simulink model "Swingup_LQR_energy_2021"  (R2021a)
settings: Solver=FixedStepAuto  StartTime=0.0  StopTime=100  RelTol=1e-3
PreLoadFcn:
  | waijung.modelPreload; % Required for working with Waijung Blockset. Do not remove.
undefined symbols (not defined in the file or in its folder): HSEOSC, Link, LQFP100, ST, STM32F407VG
libraries: simulink x2, stm32f4_io_lib x1, stm32f4_device_config_lib x1
CloseFcn:
  | waijung.modelClose; % Required for working with Waijung Blockset. Do not remove.
settings Model: Creator=MINH TAI  LastModifiedBy=NGAI-LAPTOP
settings SolverCC: AlgebraicLoopSolver=TrustRegion
settings DataIOCC: ReturnWorkspaceOutputs=off
settings OptimizationCC: DefaultParameterBehavior=Inlined  EnhancedBackFolding=on  PassReuseOutputArgsAs=Individual arguments  OptimizeBlockOrder=speed  DifferentSizesBufferReuse=on  OptimizationCustomize=off  EfficientTunableParamExpr=on
settings DebuggingCC: ParameterTunabilityLossMsg=error  SFMachineParentedDataDiag=warning  ArithmeticOperatorsInVariantConditions=warning
settings HardwareCC: ProdBitPerPointer=32  ProdBitPerSizeT=32  ProdBitPerPtrDiffT=32  ProdLargestAtomicFloat=None  ProdIntDivRoundTo=Undefined  ProdWordSize=32  ProdHWDeviceType=ARM Compatible->Cortex - M4  TargetEndianess=LittleEndian  TargetHWDeviceType=ARM Compatible->Cortex - M4
settings SFSimCC: SimUseLocalCustomCode=off  MATLABDynamicMemAlloc=off  CustomCodeUndefinedFunction=UseInterfaceOnly
settings RTWCC: Description=STM32F4 Target  SystemTargetFile=stm32f4.tlc  GenerateMakefile=off  TemplateMakefile=ert_default_tmf  GenerateReport=on  RTWUseLocalCustomCode=off  IncludeHyperlinkInReport=on  LaunchReport=on  GenerateTraceInfo=on  GenerateTraceReport=on  GenerateTraceReportSl=on  GenerateTraceReportSf=on  GenerateTraceReportEml=on  DLArmComputeVersion=20.02.1
settings CodeAppCC: ForceParamTrailComments=on  IgnoreCustomStorageClasses=off  OperatorAnnotations=on  SimulinkDataObjDesc=on  SFDataObjDesc=on  InsertBlockDesc=on
settings STFCustomTargetCC: TargetLangStandard=C99 (ISO)  MultiwordLength=256  ModelReferenceCompliant=off  CombineOutputUpdateFcns=on  ERTCustomFileBanners=on  SupportContinuousTime=off  SupportNonInlinedSFcns=off  RemoveResetFunc=on  MATLABClassNameForMDSCustomization=Simulink.SoftwareTarget.ERTCustomization  GRTInterface=off  UseToolchainInfoCompliant=off  SystemTargetFile=stm32f4.tlc
settings ERTTargetCC: TargetLangStandard=C99 (ISO)  ModelReferenceCompliant=off  ParMdlRefBuildCompliant=off  CompOptLevelCompliant=off  ConcurrentExecutionCompliant=off  ModelStepFunctionPrototypeControlCompliant=off  CPPClassGenCompliant=off  UseToolchainInfoCompliant=off  InlinedParameterPlacement=NonHierarchical  ERTSrcFileBannerTemplate=stm32f4_code_template.cgt  ERTHdrFileBannerTemplate=stm32f4_code_template.cgt  ERTDataSrcFileTemplate=stm32f4_code_template.cgt  ERTDataHdrFileTemplate=stm32f4_code_template.cgt  ERTCustomFileTemplate=stm32f4_file_process.tlc

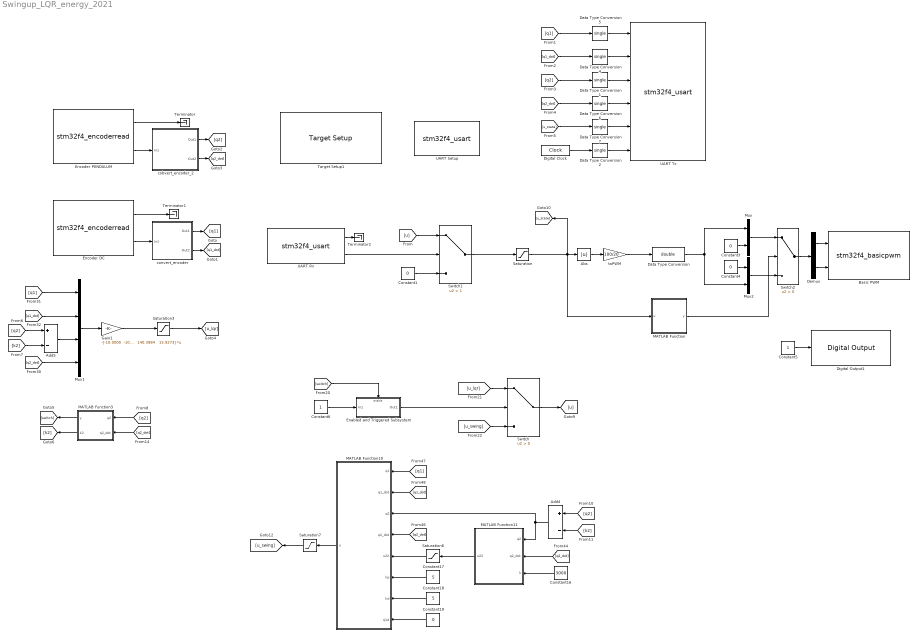
== system Swingup_LQR_energy_2021 ==
  Abs : Abs  OutDataTypeStr=single
  Add4 : Sum  Inputs=+-
  Add5 : Sum  Inputs=+-
  Basic PWM : S-Function  FunctionName=stm32f4_basicpwm  Parameters=timer,pwmperiod,ch1pin,ch2pin,ch3pin,ch4pin,sampletime,sampletimestr,blockid,apb,portstr,pinstr,pinmat,timarr,timprescale,chmat,polaritystr  SFunctionDeploymentMode=off  EnableBusSupport=off  mask(stm32f4_basicpwm){timer=4, pwmperiod=1e-3, polarity=Active High, polaritystr=TIM_OCPolarity_High, ch1pin=Not available - Do not use, ch2pin=D13, ch3pin=Not available - Do not use, ch4pin=D15, sampletime=0.02, sampletimestr=-1, blockid=BasicPWM, portpinstr=,D13,,D15, enablecustomportlabel=off, cinputportlabel=In1, In2, In3, In4, coutputportlabel=0, apb=1, portstr=["D"], pinstr=["GPIO_Pin_13 | GPIO_Pin_15"], pinmat=[2 13 15], timarr=41999, timprescale=1, chmat=[2  4]}
      mask prompts: pwmperiod "PWM Period (seconds)"; ch1pin "Channel 1"; ch2pin "Channel 2"; ch3pin "Channel 3"; ch4pin "Channel 4"; sampletime "Sample time (sec)"; sampletimestr "Compiled sample time (sec) in string"; portpinstr "Port pin string"; enablecustomportlabel "Enable custom port labels"; cinputportlabel "Custom input port labels (Ex. In1, In2, In3)"; coutputportlabel "Custom output port labels (Ex. Out1, Out2, Out3)"; portstr "Port string"; pinstr "Pin string"; pinmat "Pin matrix"; timarr "Timer ARR"; timprescale "Timer PRESCALE"; chmat "Channel order"
      mask help:
      | This block implements basic Edge-aligned Pulse Width Modulation (PWM) generation.
      | All timers are 16-bit. The PWM period is fixed (per timer).
      mask init:
      | stm32f4_basicpwm_callback('init');
      mask Help: web(fullfile(waijungdocroot,'stm32f4_basicpwm.htm'),'-browser')
      mask TypeOptions timer: 1 | 2 | 3 | 4 | 5 | 8 | 9 | 10 | 11 | 12 | 13 | 14
      mask Callback timer: stm32f4_basicpwm_callback('timer');
      mask Callback pwmperiod: stm32f4_basicpwm_callback('pwmperiod');
      mask TypeOptions polarity: Active High | Active Low
      mask Callback polarity: stm32f4_basicpwm_callback('polarity');
      mask TypeOptions ch1pin: Not available - Do not use | B6 | D12
      mask Callback ch1pin: stm32f4_basicpwm_callback('ch1pin');
      mask TypeOptions ch2pin: Not available - Do not use | B7 | D13
      mask Callback ch2pin: stm32f4_basicpwm_callback('ch2pin');
      mask TypeOptions ch3pin: Not available - Do not use | B8 | D14
      mask Callback ch3pin: stm32f4_basicpwm_callback('ch3pin');
      mask TypeOptions ch4pin: Not available - Do not use | B9 | D15
      mask Callback ch4pin: stm32f4_basicpwm_callback('ch4pin');
      mask Callback sampletime: stm32f4_basicpwm_callback('sampletime');
      mask Callback sampletimestr: stm32f4_basicpwm_callback('sampletimestr');
      mask Callback blockid: stm32f4_basicpwm_callback('blockid');
      mask Callback enablecustomportlabel: stm32f4_basicpwm_callback('enablecustomportlabel');
      mask Display: text(0.95, 0.5, 'Timer: 4\nPolarity: Active High\nPeriod (sec) 1e-3\nTs (sec): -1','ver','middle','hor','right');port_label('input', 1,'CH2 (D13)');port_label('input', 2,'CH4 (D15)')
  Constant1 : Constant  Value=0  SampleTime=0.02
  Constant16 : Constant  Value=3000  SampleTime=-1
  Constant17 : Constant  Value=5  SampleTime=-1
  Constant18 : Constant  Value=5  SampleTime=-1
  Constant19 : Constant  Value=0  SampleTime=-1
  Constant3 : Constant  Value=0  SampleTime=0.02
  Constant4 : Constant  Value=0  SampleTime=0.02
  Constant5 : Constant  SampleTime=0.02
  Constant6 : Constant  SampleTime=0.02
  Data Type Conversion : DataTypeConversion  OutDataTypeStr=double
  Data Type Conversion{1..2,4..7} (6 alike) : DataTypeConversion  OutDataTypeStr=single
  Demux : Demux  Outputs=2
  Digital Clock : DigitalClock  SampleTime=0.02
  Digital Output1 : stm32f4_io_lib/Digital Output  use_bitband=on  port=D  speed=100  porttype=Push Pull  porttypestr=PP  use_pin0=off  use_pin1=off  use_pin2=off  use_pin3=off  use_pin4=off  use_pin5=off  use_pin6=off  use_pin7=off  use_pin8=off  use_pin9=off  use_pin10=off  use_pin11=off  use_pin12=off  use_pin13=off  use_pin14=on  use_pin15=off  pinstr=GPIO_Pin_14  usedpinarray="[0  0  0  0  0  0  0  0  0  0  0  0  0  0  1  0]"  bitbandingstr="#define DigitalOutput1_D14 Peripheral_BB(GPIOD->ODR, 14)  /* Output pin */"  sampletime=-1  sampletimestr=-1  blockid=DigitalOutput1  enablecustomportlabel=off  globalinit=off  cinputportlabel=In1, In2  coutputportlabel=0
      settings: SourceProductName=Waijung Blockset
  Enabled and Triggered Subsystem : Subsystem  TreatAsAtomicUnit=on
  Encoder DC : S-Function  FunctionName=stm32f4_encoderread  Parameters=sampletime,sampletimestr,blockid,timer,apb,portstr,pinstr,pinmat,chmat,filterstr,filter,factor,rstcnt,ppr  SFunctionDeploymentMode=off  EnableBusSupport=off  mask(stm32f4_encoderread){timer=3, ch1=B4, ch2=B5, ppr=65535, rstcnt=off, filterstr=No filter; sampling is done at fDTS, sampletime=0.02, sampletimestr=-1, blockid=EncoderDC, absresetinput=off, portpinstr=B4,B5, portstr=["B"], pinstr=["GPIO_Pin_4 | GPIO_Pin_5"], pinmat=[2 4 5], chmat=[1  2], apb=1, filter=0, factor=4}
      mask prompts: ch1 "Channel A Input Pin"; ch2 "Channel B Input Pin"; ppr "PPR (Number of pulses generated per revolution)"; rstcnt "Reset counter after every counter read"; filterstr "Built-in Input Capture Filter"; sampletime "Sample time (sec)"; sampletimestr "Compiled sample time (sec) in string"; absresetinput "Enable absolute position reset input signal"; portpinstr "Port pin string"; portstr "Port string"; pinstr "Pin string"; pinmat "Pin matrix"; chmat "Channel order"; filter "Filter ID"
      mask help:
      | The output Direction (uint32) is the direction of rotation either 0 or 1.
      |
      | The output Position (count) (uint32) is the count of number of edges of the encoder output signals from either channel A and B. The decoder is set to count at every rising and falling edge of both channel A and B (4x) or (x2) for one channel. For example, if an encoder has 180 pulses per revolution (PPS) and two channels are selected, the maximum count is 720 per revolution (4x180 = 720), i.e. from 0 to 719.
      mask init:
      | stm32f4_encoderread_callback('init');
      mask Help: web(fullfile(waijungdocroot,'stm32f4_encoderread.htm'),'-browser')
      mask TypeOptions timer: 1 | 2 | 3 | 4 | 5 | 8
      mask Callback timer: stm32f4_encoderread_callback('timer');
      mask TypeOptions ch1: Not available - Do not use | A6 | B4 | C6
      mask Callback ch1: stm32f4_encoderread_callback('chA');
      mask TypeOptions ch2: Not available - Do not use | A7 | B5 | C7
      mask Callback ch2: stm32f4_encoderread_callback('chB');
      mask Callback ppr: stm32f4_encoderread_callback('ppr');
      mask Callback rstcnt: stm32f4_encoderread_callback('rstcnt');
      mask TypeOptions filterstr: No filter; sampling is done at fDTS | fSAMPLING=fCK_INT; N=2 | fSAMPLING=fCK_INT; N=4 | fSAMPLING=fCK_INT; N=8 | fSAMPLING=fDTS/2; N=6 | fSAMPLING=fDTS/2; N=8 | fSAMPLING=fDTS/4; N=6 | fSAMPLING=fDTS/4; N=8 | fSAMPLING=fDTS/8; N=6 | fSAMPLING=fDTS/8; N=8 | fSAMPLING=fDTS/16; N=5 | fSAMPLING=fDTS/16; N=6 | fSAMPLING=fDTS/16; N=8 | fSAMPLING=fDTS/32; N=5 | fSAMPLING=fDTS/32; N=6 | fSAMPLING=fDTS/32; N=8
      mask Callback filterstr: stm32f4_encoderread_callback('filterstr');
      mask Callback sampletimestr: stm32f4_encoderread_callback('sampletimestr');
      mask Callback blockid: stm32f4_encoderread_callback('blockid');
      mask Display: text(0.05, 0.5, 'Timer: 3\nInput pins [CH_A, CH_B]: [B4,B5]\nRST Counter: No\nTs (sec): -1','ver','middle','hor','left');port_label('output', 1, 'Direction');port_label('output', 2, 'Position (count)')
  Encoder PENDULUM : S-Function  FunctionName=stm32f4_encoderread  Parameters=sampletime,sampletimestr,blockid,timer,apb,portstr,pinstr,pinmat,chmat,filterstr,filter,factor,rstcnt,ppr  SFunctionDeploymentMode=off  EnableBusSupport=off  mask(stm32f4_encoderread){timer=1, ch1=E9, ch2=E11, ppr=65535, rstcnt=off, filterstr=No filter; sampling is done at fDTS, sampletime=0.02, sampletimestr=-1, blockid=EncoderPENDULUM, absresetinput=off, portpinstr=E9,E11, portstr=["E"], pinstr=["GPIO_Pin_9 | GPIO_Pin_11"], pinmat=[2 9 11], chmat=[1  2], apb=2, filter=0, factor=4}
      mask prompts: ch1 "Channel A Input Pin"; ch2 "Channel B Input Pin"; ppr "PPR (Number of pulses generated per revolution)"; rstcnt "Reset counter after every counter read"; filterstr "Built-in Input Capture Filter"; sampletime "Sample time (sec)"; sampletimestr "Compiled sample time (sec) in string"; absresetinput "Enable absolute position reset input signal"; portpinstr "Port pin string"; portstr "Port string"; pinstr "Pin string"; pinmat "Pin matrix"; chmat "Channel order"; filter "Filter ID"
      mask help:
      | The output Direction (uint32) is the direction of rotation either 0 or 1.
      |
      | The output Position (count) (uint32) is the count of number of edges of the encoder output signals from either channel A and B. The decoder is set to count at every rising and falling edge of both channel A and B (4x) or (x2) for one channel. For example, if an encoder has 180 pulses per revolution (PPS) and two channels are selected, the maximum count is 720 per revolution (4x180 = 720), i.e. from 0 to 719.
      mask init:
      | stm32f4_encoderread_callback('init');
      mask Help: web(fullfile(waijungdocroot,'stm32f4_encoderread.htm'),'-browser')
      mask TypeOptions timer: 1 | 2 | 3 | 4 | 5 | 8
      mask Callback timer: stm32f4_encoderread_callback('timer');
      mask TypeOptions ch1: Not available - Do not use | E9 | A8
      mask Callback ch1: stm32f4_encoderread_callback('chA');
      mask TypeOptions ch2: Not available - Do not use | E11 | A9
      mask Callback ch2: stm32f4_encoderread_callback('chB');
      mask Callback ppr: stm32f4_encoderread_callback('ppr');
      mask Callback rstcnt: stm32f4_encoderread_callback('rstcnt');
      mask TypeOptions filterstr: No filter; sampling is done at fDTS | fSAMPLING=fCK_INT; N=2 | fSAMPLING=fCK_INT; N=4 | fSAMPLING=fCK_INT; N=8 | fSAMPLING=fDTS/2; N=6 | fSAMPLING=fDTS/2; N=8 | fSAMPLING=fDTS/4; N=6 | fSAMPLING=fDTS/4; N=8 | fSAMPLING=fDTS/8; N=6 | fSAMPLING=fDTS/8; N=8 | fSAMPLING=fDTS/16; N=5 | fSAMPLING=fDTS/16; N=6 | fSAMPLING=fDTS/16; N=8 | fSAMPLING=fDTS/32; N=5 | fSAMPLING=fDTS/32; N=6 | fSAMPLING=fDTS/32; N=8
      mask Callback filterstr: stm32f4_encoderread_callback('filterstr');
      mask Callback sampletimestr: stm32f4_encoderread_callback('sampletimestr');
      mask Callback blockid: stm32f4_encoderread_callback('blockid');
      mask Display: text(0.05, 0.5, 'Timer: 1\nInput pins [CH_A, CH_B]: [E9,E11]\nRST Counter: No\nTs (sec): -1','ver','middle','hor','left');port_label('output', 1, 'Direction');port_label('output', 2, 'Position (count)')
  Gain1 : Gain  Gain="-[-10.0000  -10.0487  140.3984   15.9273]"  Multiplication=Matrix(K*u)
  MATLAB Function : MATLAB Function  TreatAsAtomicUnit=on
  MATLAB Function10 : MATLAB Function  TreatAsAtomicUnit=on
  MATLAB Function11 : MATLAB Function  TreatAsAtomicUnit=on
  MATLAB Function3 : MATLAB Function  TreatAsAtomicUnit=on
  Mux : Mux  Inputs=2
  Mux1 : Mux
  Mux2 : Mux  Inputs=2
  Saturation : Saturate  UpperLimit=12  LowerLimit=-12
  Saturation3 : Saturate  UpperLimit=10  LowerLimit=-10
  Saturation6 : Saturate  UpperLimit=5  LowerLimit=-5  LinearizeAsGain=off
  Saturation7 : Saturate  UpperLimit=12  LowerLimit=-12
  Switch : Switch  Criteria=u2 > Threshold
  Switch1 : Switch  Criteria=u2 > Threshold  Threshold=1
  Switch2 : Switch  Criteria=u2 > Threshold
  Target Setup1 : stm32f4_device_config_lib/Target Setup  Priority=100  compiler=GNU ARM  previous_compiler=GNU ARM  mcu=STM32F407VG (LQFP100)  mcustr=STM32F407VG  clockconfig=HSEOSC-8MHz  system_stm32f4xx_c_path=E:\2024\MATLAB_STM32F4\waijung18_11a_2\waijung_18.11a\targets\stm32f4_target\stm32f4\utils\system_stm32f4xx_default\STM32F40_41xxx\hseosc8mhz  showmemoryconfiguration=off  stacksize=0x2000  heapsize=0x2000  enableautocompiledownload=on  fullchiperase=on  programmerinterface=ST-Link  editctrlstr=off  compilercontrolstr=$(patsubst %, -I%, .) -mcpu=cortex-m4 -mthumb -mthumb-interwork -mfloat-abi=hard -mfpu=fpv4-sp-d16 -ffast-math -Wall -Wextra -Ofast  assemblercontrolstr=$(patsubst %, -I%, .) -mcpu=cortex-m4 -mthumb -mthumb-interwork -mfloat-abi=hard -mfpu=fpv4-sp-d16 -ffast-math -Wall -Wextra -Ofast -Wa,-amhls=$(<:.s=.lst) -D__STACK_SIZE=$(STACK_SIZE) -D__HEAP_SIZE=$(HEAP_SIZE)  linkercontrolstr=-T$(LD_SCRIPT) -g -Wl,-Map=$(MAP),--cref,--no-warn-mismatch -mcpu=cortex-m4 -mthumb -mthumb-interwork -mfloat-abi=hard -mfpu=fpv4-sp-d16 -specs=nosys.specs  runafterdownload=on  execprofile=None  profileruart=3  profilerbaud=500000  profilertxpin=D8  profilerinitstr=0.01,168000000,1680000,500000,0  manualsetsampletime=on  sampletime=0.01  blockid=TargetSetup1  systickreloadvalue=1680000  hseval=8000000  lastprofileruart=3  hclk=168000000  flashorigin=0x8000000  flashlength=1024k  ramorigin=0x20000000  ramlength=128k  useextram=off
      settings: SourceProductName=Waijung Blockset
  Terminator : Terminator
  Terminator1 : Terminator
  Terminator2 : Terminator
  UART Rx : S-Function  Priority=1  FunctionName=stm32f4_usart  Parameters=configuration,uartmodule,transfer,baudrate,inputtype,outputtype,confstr,binheaderarray,binterminatorarray,asciiheader,asciiterminator,bindatalength,packetmode,varname,sampletime,sampletimestr,blockid  SFunctionDeploymentMode=off  EnableBusSupport=off  mask(stm32f4_usart){configuration=Rx, uartmodule=3, baudrate=115200, databits=8, parity=No, stopbit=1, remaptxpin=Not used, remaprxpin=Not used, flowcontrol=None, remapctspin=Not used, remaprtspin=Not used, advanceoptions=off, rxbuffersize=512, txbuffersize=512, transfer=Non-Blocking, packetmode=Ascii, binheader='7E 7E', binterminator='03 03', porttype_double=1, porttype_single=0, porttype_int8=1, porttype_uint8=0, porttype_int16=0, porttype_uint16=0, porttype_int32=0, porttype_uint32=0, asciiformat='%u', rx_asciiterminator=CRLF (0x0D 0x0A - "\r\n"), tx_asciiterminator=LF (0x0A - "\n"), storagename=<empty>, varname=, inputtype=[0], outputtype=[2 3  7], binheaderarray=[0], binterminatorarray=[0], bindatalength=0, asciiheader='%u\r\n', asciiterminator=[2 13 10], sampletime=0.02, sampletimestr=-1, blockid=UARTRx, confstr=[ "dummy", "0", "*", "*", "0", "*", "*", "0", "*", "*", "0", "*", "*", "1", "4", "3", "1", "4", "1", "512", "512", "1", "3", "115200", "8", "No", "1", "None", "USART3"], lastmodule=1}
      mask prompts: uartmodule "UART Module"; baudrate "Baud rate (bps)"; databits "Data bits"; stopbit "Stop bit"; remaptxpin "Tx Pin"; remaprxpin "Rx Pin"; flowcontrol "Hardware flow control"; remapctspin "HW Flow control, CTS Pin"; remaprtspin "HW Flow control, RTS Pin"; advanceoptions "Advance options"; rxbuffersize "Rx buffer size (bytes)"; txbuffersize "Tx buffer size (bytes)"; packetmode "Packet mode"; binheader "Binary header (example: '7E 7E')"; binterminator "Binary terminator (example: '03 03')"; porttype_double "Number of data port, type DOUBLE"; porttype_single "Number of data port, type SINGLE"; porttype_int8 "Number of data port, type INT8"; porttype_uint8 "Number of data port, type UINT8"; porttype_int16 "Number of data port, type INT16"; porttype_uint16 "Number of data port, type UINT16"; porttype_int32 "Number of data port, type INT32"; porttype_uint32 "Number of data port, type UINT32"; asciiformat "Ascii format"; rx_asciiterminator "End of packet"; tx_asciiterminator "End of packet"; storagename "Buffer"; varname "Var name"; inputtype "Input data type"; outputtype "Output data type"; binheaderarray "Binary header"; binterminatorarray "Binary terminator"; bindatalength "Binary data length"; asciiheader "Ascii header (printf format)"; asciiterminator "Ascii terminator"; sampletime "Sample time (sec)"; sampletimestr "Compiled sample time (sec) in string"; confstr "Configuration string"; lastmodule "Last module selected"
      mask help:
      | Data type for Ascii format
      | %u, %i, %d, %o, %x: uint32
      | %e, %g, %f: single
      | %c: int8
      mask init:
      | stm32f4_usart_callback('init');
      mask Help: web(fullfile(waijungdocroot,'stm32f4_usart_rx.htm'), '-browser')
      mask TypeOptions configuration: Setup | Tx | Rx
      mask Callback configuration: stm32f4_usart_callback('configuration');
      mask TypeOptions uartmodule: 1 | 2 | 3 | 4 | 5 | 6
      mask Callback uartmodule: stm32f4_usart_callback('uartmodule');
      mask Callback baudrate: stm32f4_usart_callback('baudrate');
      mask TypeOptions databits: 8
      mask TypeOptions parity: No | Odd | Even
      mask TypeOptions stopbit: 0.5 | 1 | 1.5 | 2
      mask TypeOptions remaptxpin: Not used | A9 | B6
      mask TypeOptions remaprxpin: Not used | A10 | B7
      mask TypeOptions flowcontrol: None | RTS | CTS | RTS/CTS
      mask Callback flowcontrol: stm32f4_usart_callback('flowcontrol');
      mask TypeOptions remapctspin: Not used | A11
      mask TypeOptions remaprtspin: Not used | A12
      mask Callback advanceoptions: stm32f4_usart_callback('advanceoptions');
      mask TypeOptions rxbuffersize: 16 | 32 | 64 | 128 | 256 | 512 | 1024 | 2048
      mask TypeOptions txbuffersize: 16 | 32 | 64 | 128 | 256 | 512 | 1024 | 2048
      mask TypeOptions transfer: Blocking | Non-Blocking
      mask Callback transfer: stm32f4_usart_callback('transfer');
      mask TypeOptions packetmode: Ascii | Binary | Binary Vector | String Buffer | Raw Buffer | Read Line
      mask Callback packetmode: stm32f4_usart_callback('packetmode');
      mask Callback binheader: stm32f4_usart_callback('binheader');
      mask Callback binterminator: stm32f4_usart_callback('binterminator');
      mask Callback porttype_double: stm32f4_usart_callback('porttype');
      mask Callback porttype_single: stm32f4_usart_callback('porttype');
      mask Callback porttype_int8: stm32f4_usart_callback('porttype');
      mask Callback porttype_uint8: stm32f4_usart_callback('porttype');
      mask Callback porttype_int16: stm32f4_usart_callback('porttype');
      mask Callback porttype_uint16: stm32f4_usart_callback('porttype');
      mask Callback porttype_int32: stm32f4_usart_callback('porttype');
      mask Callback porttype_uint32: stm32f4_usart_callback('porttype');
      mask Callback asciiformat: stm32f4_usart_callback('asciiformat');
      mask TypeOptions rx_asciiterminator: CR (0x0D - "\r") | LF (0x0A - "\n") | CRLF (0x0D 0x0A - "\r\n")
      mask Callback rx_asciiterminator: stm32f4_usart_callback('rx_asciiterminator');
      mask TypeOptions tx_asciiterminator: CR (0x0D - "\r") | LF (0x0A - "\n") | CRLF (0x0D 0x0A - "\r\n") | None
      mask Callback tx_asciiterminator: stm32f4_usart_callback('tx_asciiterminator');
      mask TypeOptions storagename: <empty>
      mask Callback storagename: stm32f4_usart_callback('storagename');
      mask Callback varname: stm32f4_usart_callback('varname');
      mask Callback sampletime: stm32f4_usart_callback('sampletime');
      mask Callback sampletimestr: stm32f4_usart_callback('sampletimestr');
      mask Callback blockid: stm32f4_usart_callback('blockid');
      mask Display: text(0.05, 0.5, 'Module: USART3_Rx\nPacket: Ascii\nTransfer: Non-Blocking\nTs (sec): -1','ver','middle','hor','left'); port_label('output', 1,'READY'); port_label('output', 2,'uint32');
  UART Setup : S-Function  Priority=1  FunctionName=stm32f4_usart  Parameters=configuration,uartmodule,transfer,baudrate,inputtype,outputtype,confstr,binheaderarray,binterminatorarray,asciiheader,asciiterminator,bindatalength,packetmode,varname,sampletime,sampletimestr,blockid  SFunctionDeploymentMode=off  EnableBusSupport=off  mask(stm32f4_usart){configuration=Setup, uartmodule=3, baudrate=115200, databits=8, parity=No, stopbit=1, remaptxpin=D8, remaprxpin=D9, flowcontrol=None, remapctspin=Not used, remaprtspin=Not used, advanceoptions=off, rxbuffersize=512, txbuffersize=512, transfer=Blocking, packetmode=Ascii, binheader='7E 7E', binterminator='03 03', porttype_double=1, porttype_single=0, porttype_int8=1, porttype_uint8=0, porttype_int16=0, porttype_uint16=0, porttype_int32=0, porttype_uint32=0, asciiformat='%d,%f', rx_asciiterminator=CRLF (0x0D 0x0A - "\r\n"), tx_asciiterminator=CR (0x0D - "\r"), storagename=<empty>, varname=, inputtype=[0], outputtype=[0], binheaderarray=[0], binterminatorarray=[0], bindatalength=0, asciiheader='', asciiterminator=[0], sampletime=-1, sampletimestr=-1, blockid=UARTSetup, confstr=[ "dummy", "1", "D", "8", "1", "D", "9", "0", "*", "*", "0", "*", "*", "1", "4", "3", "1", "4", "1", "512", "512", "1", "3", "115200", "8", "No", "1", "None", "USART3"], lastmodule=3}
      mask prompts: uartmodule "UART Module"; baudrate "Baud rate (bps)"; databits "Data bits"; stopbit "Stop bit"; remaptxpin "Tx Pin"; remaprxpin "Rx Pin"; flowcontrol "Hardware flow control"; remapctspin "HW Flow control, CTS Pin"; remaprtspin "HW Flow control, RTS Pin"; advanceoptions "Advance options"; rxbuffersize "Rx buffer size (bytes)"; txbuffersize "Tx buffer size (bytes)"; packetmode "Packet mode"; binheader "Binary header (example: '7E 7E')"; binterminator "Binary terminator (example: '03 03')"; porttype_double "Number of data port, type DOUBLE"; porttype_single "Number of data port, type SINGLE"; porttype_int8 "Number of data port, type INT8"; porttype_uint8 "Number of data port, type UINT8"; porttype_int16 "Number of data port, type INT16"; porttype_uint16 "Number of data port, type UINT16"; porttype_int32 "Number of data port, type INT32"; porttype_uint32 "Number of data port, type UINT32"; asciiformat "Ascii format"; rx_asciiterminator "End of packet"; tx_asciiterminator "End of packet"; storagename "Buffer"; varname "Var name"; inputtype "Input data type"; outputtype "Output data type"; binheaderarray "Binary header"; binterminatorarray "Binary terminator"; bindatalength "Binary data length"; asciiheader "Ascii header (printf format)"; asciiterminator "Ascii terminator"; sampletime "Sample time (sec)"; sampletimestr "Compiled sample time (sec) in string"; confstr "Configuration string"; lastmodule "Last module selected"
      mask help:
      | Default STM32F4DISCOVERY + aMG F4 Connect 2 + aMG USB Converter N2 settings use
      |
      | USART3, Tx D8, Rx D9 and USB Serial Converter A.
      mask init:
      | stm32f4_usart_callback('init');
      mask Help: web(fullfile(waijungdocroot,'stm32f4_usart_setup.htm'), '-browser')
      mask TypeOptions configuration: Setup | Tx | Rx
      mask Callback configuration: stm32f4_usart_callback('configuration');
      mask TypeOptions uartmodule: 1 | 2 | 3 | 4 | 5 | 6
      mask Callback uartmodule: stm32f4_usart_callback('uartmodule');
      mask Callback baudrate: stm32f4_usart_callback('baudrate');
      mask TypeOptions databits: 8
      mask TypeOptions parity: No | Odd | Even
      mask TypeOptions stopbit: 0.5 | 1 | 1.5 | 2
      mask TypeOptions remaptxpin: Not used | B10 | C10 | D8
      mask TypeOptions remaprxpin: Not used | B11 | C11 | D9
      mask TypeOptions flowcontrol: None | RTS | CTS | RTS/CTS
      mask Callback flowcontrol: stm32f4_usart_callback('flowcontrol');
      mask TypeOptions remapctspin: Not used | B13 | D11
      mask TypeOptions remaprtspin: Not used | B14 | D12
      mask Callback advanceoptions: stm32f4_usart_callback('advanceoptions');
      mask TypeOptions rxbuffersize: 16 | 32 | 64 | 128 | 256 | 512 | 1024 | 2048
      mask TypeOptions txbuffersize: 16 | 32 | 64 | 128 | 256 | 512 | 1024 | 2048
      mask TypeOptions transfer: Blocking | Non-Blocking
      mask Callback transfer: stm32f4_usart_callback('transfer');
      mask TypeOptions packetmode: Ascii | Binary | String Buffer
      mask Callback packetmode: stm32f4_usart_callback('packetmode');
      mask Callback binheader: stm32f4_usart_callback('binheader');
      mask Callback binterminator: stm32f4_usart_callback('binterminator');
      mask Callback porttype_double: stm32f4_usart_callback('porttype');
      mask Callback porttype_single: stm32f4_usart_callback('porttype');
      mask Callback porttype_int8: stm32f4_usart_callback('porttype');
      mask Callback porttype_uint8: stm32f4_usart_callback('porttype');
      mask Callback porttype_int16: stm32f4_usart_callback('porttype');
      mask Callback porttype_uint16: stm32f4_usart_callback('porttype');
      mask Callback porttype_int32: stm32f4_usart_callback('porttype');
      mask Callback porttype_uint32: stm32f4_usart_callback('porttype');
      mask Callback asciiformat: stm32f4_usart_callback('asciiformat');
      mask TypeOptions rx_asciiterminator: CR (0x0D - "\r") | LF (0x0A - "\n") | CRLF (0x0D 0x0A - "\r\n")
      mask Callback rx_asciiterminator: stm32f4_usart_callback('rx_asciiterminator');
      mask TypeOptions tx_asciiterminator: CR (0x0D - "\r") | LF (0x0A - "\n") | CRLF (0x0D 0x0A - "\r\n") | None
      mask Callback tx_asciiterminator: stm32f4_usart_callback('tx_asciiterminator');
      mask TypeOptions storagename: <empty>
      mask Callback storagename: stm32f4_usart_callback('storagename');
      mask Callback varname: stm32f4_usart_callback('varname');
      mask Callback sampletime: stm32f4_usart_callback('sampletime');
      mask Callback sampletimestr: stm32f4_usart_callback('sampletimestr');
      mask Callback blockid: stm32f4_usart_callback('blockid');
      mask Display: text(0.5, 0.5, 'Module: USART3_Setup\nBaud (Bps): 115200\nDMA Buffer: 512/512\nTx/Rx Pin: D8/D9','ver','middle','hor','center');
  UART Tx : S-Function  Priority=1  FunctionName=stm32f4_usart  Parameters=configuration,uartmodule,transfer,baudrate,inputtype,outputtype,confstr,binheaderarray,binterminatorarray,asciiheader,asciiterminator,bindatalength,packetmode,varname,sampletime,sampletimestr,blockid  SFunctionDeploymentMode=off  EnableBusSupport=off  mask(stm32f4_usart){configuration=Tx, uartmodule=3, baudrate=115200, databits=8, parity=No, stopbit=1, remaptxpin=Not used, remaprxpin=Not used, flowcontrol=None, remapctspin=Not used, remaprtspin=Not used, advanceoptions=off, rxbuffersize=512, txbuffersize=512, transfer=Blocking, packetmode=Ascii, binheader='7E 7E', binterminator='03 03', porttype_double=1, porttype_single=0, porttype_int8=1, porttype_uint8=0, porttype_int16=0, porttype_uint16=0, porttype_int32=0, porttype_uint32=0, asciiformat='%f, %f, %f, %f, %f, %f', rx_asciiterminator=CRLF (0x0D 0x0A - "\r\n"), tx_asciiterminator=LF (0x0A - "\n"), storagename=<empty>, varname=, inputtype=[6  1 1 1 1 1 1], outputtype=[0], binheaderarray=[0], binterminatorarray=[0], bindatalength=0, asciiheader='%f, %f, %f, %f, %f, %f\n', asciiterminator=[1 10], sampletime=-1, sampletimestr=-1, blockid=UARTTx, confstr=[ "dummy", "0", "*", "*", "0", "*", "*", "0", "*", "*", "0", "*", "*", "1", "4", "3", "1", "4", "1", "512", "512", "1", "3", "115200", "8", "No", "1", "None", "USART3"], lastmodule=1}
      mask prompts: uartmodule "UART Module"; baudrate "Baud rate (bps)"; databits "Data bits"; stopbit "Stop bit"; remaptxpin "Tx Pin"; remaprxpin "Rx Pin"; flowcontrol "Hardware flow control"; remapctspin "HW Flow control, CTS Pin"; remaprtspin "HW Flow control, RTS Pin"; advanceoptions "Advance options"; rxbuffersize "Rx buffer size (bytes)"; txbuffersize "Tx buffer size (bytes)"; packetmode "Packet mode"; binheader "Binary header (example: '7E 7E')"; binterminator "Binary terminator (example: '03 03')"; porttype_double "Number of data port, type DOUBLE"; porttype_single "Number of data port, type SINGLE"; porttype_int8 "Number of data port, type INT8"; porttype_uint8 "Number of data port, type UINT8"; porttype_int16 "Number of data port, type INT16"; porttype_uint16 "Number of data port, type UINT16"; porttype_int32 "Number of data port, type INT32"; porttype_uint32 "Number of data port, type UINT32"; asciiformat "Ascii format"; rx_asciiterminator "End of packet"; tx_asciiterminator "End of packet"; storagename "Buffer"; varname "Var name"; inputtype "Input data type"; outputtype "Output data type"; binheaderarray "Binary header"; binterminatorarray "Binary terminator"; bindatalength "Binary data length"; asciiheader "Ascii header (printf format)"; asciiterminator "Ascii terminator"; sampletime "Sample time (sec)"; sampletimestr "Compiled sample time (sec) in string"; confstr "Configuration string"; lastmodule "Last module selected"
      mask help:
      | Data type for Ascii format
      | %u, %i, %d, %o, %x: uint32
      | %e, %g, %f: single
      | %c: int8
      mask init:
      | stm32f4_usart_callback('init');
      mask Help: web(fullfile(waijungdocroot,'stm32f4_usart_tx.htm'), '-browser')
      mask TypeOptions configuration: Setup | Tx | Rx
      mask Callback configuration: stm32f4_usart_callback('configuration');
      mask TypeOptions uartmodule: 1 | 2 | 3 | 4 | 5 | 6
      mask Callback uartmodule: stm32f4_usart_callback('uartmodule');
      mask Callback baudrate: stm32f4_usart_callback('baudrate');
      mask TypeOptions databits: 8
      mask TypeOptions parity: No | Odd | Even
      mask TypeOptions stopbit: 0.5 | 1 | 1.5 | 2
      mask TypeOptions remaptxpin: Not used | A9 | B6
      mask TypeOptions remaprxpin: Not used | A10 | B7
      mask TypeOptions flowcontrol: None | RTS | CTS | RTS/CTS
      mask Callback flowcontrol: stm32f4_usart_callback('flowcontrol');
      mask TypeOptions remapctspin: Not used | A11
      mask TypeOptions remaprtspin: Not used | A12
      mask Callback advanceoptions: stm32f4_usart_callback('advanceoptions');
      mask TypeOptions rxbuffersize: 16 | 32 | 64 | 128 | 256 | 512 | 1024 | 2048
      mask TypeOptions txbuffersize: 16 | 32 | 64 | 128 | 256 | 512 | 1024 | 2048
      mask TypeOptions transfer: Blocking | Non-Blocking
      mask Callback transfer: stm32f4_usart_callback('transfer');
      mask TypeOptions packetmode: Ascii | Binary | Binary Vector | String Buffer | Raw Buffer
      mask Callback packetmode: stm32f4_usart_callback('packetmode');
      mask Callback binheader: stm32f4_usart_callback('binheader');
      mask Callback binterminator: stm32f4_usart_callback('binterminator');
      mask Callback porttype_double: stm32f4_usart_callback('porttype');
      mask Callback porttype_single: stm32f4_usart_callback('porttype');
      mask Callback porttype_int8: stm32f4_usart_callback('porttype');
      mask Callback porttype_uint8: stm32f4_usart_callback('porttype');
      mask Callback porttype_int16: stm32f4_usart_callback('porttype');
      mask Callback porttype_uint16: stm32f4_usart_callback('porttype');
      mask Callback porttype_int32: stm32f4_usart_callback('porttype');
      mask Callback porttype_uint32: stm32f4_usart_callback('porttype');
      mask Callback asciiformat: stm32f4_usart_callback('asciiformat');
      mask TypeOptions rx_asciiterminator: CR (0x0D - "\r") | LF (0x0A - "\n") | CRLF (0x0D 0x0A - "\r\n")
      mask Callback rx_asciiterminator: stm32f4_usart_callback('rx_asciiterminator');
      mask TypeOptions tx_asciiterminator: CR (0x0D - "\r") | LF (0x0A - "\n") | CRLF (0x0D 0x0A - "\r\n") | None
      mask Callback tx_asciiterminator: stm32f4_usart_callback('tx_asciiterminator');
      mask TypeOptions storagename: <empty>
      mask Callback storagename: stm32f4_usart_callback('storagename');
      mask Callback varname: stm32f4_usart_callback('varname');
      mask Callback sampletime: stm32f4_usart_callback('sampletime');
      mask Callback sampletimestr: stm32f4_usart_callback('sampletimestr');
      mask Callback blockid: stm32f4_usart_callback('blockid');
      mask Display: text(0.95, 0.5, 'Module: USART3_Tx\nPacket: Ascii\nTransfer: Blocking\nTs (sec): -1','ver','middle','hor','right'); port_label('input', 1,'single'); port_label('input', 2,'single'); port_label('input', 3,'single'); port_label('input', 4,'single'); port_label('input', 5,'single'); port_label('input', 6,'single');
  cobvert_encoder_2 : Subsystem
  convert_encoder : Subsystem
  toPWM : Gain  Gain=100/20  ParamDataTypeStr=single  OutDataTypeStr=single
  wires:
  toPWM/1 -> Data Type Conversion/1
  Abs/1 -> toPWM/1
  Data Type Conversion4/1 -> UART Tx/2
  Data Type Conversion5/1 -> UART Tx/1
  Data Type Conversion7/1 -> UART Tx/5
  Data Type Conversion6/1 -> UART Tx/4
  Data Type Conversion1/1 -> UART Tx/3
  [q1] -> Data Type Conversion5/1
  [q1_dot] -> Data Type Conversion4/1
  [q2] -> Data Type Conversion1/1
  [q2_dot] -> Data Type Conversion6/1
  [u_state] -> Data Type Conversion7/1
  Switch1/1 -> Saturation/1
  Encoder PENDULUM/1 -> Terminator/1
  Encoder DC/1 -> Terminator1/1
  MATLAB Function3/1(y) -> [switch]
  MATLAB Function3/2(k2) -> [k2]
  [q2_dot] -> MATLAB Function3/2(q2_dot)
  Switch/1 -> [u]
  Constant1/1 -> Switch1/3
  UART Rx/2 -> Switch1/2
  UART Rx/1 -> Terminator2/1
  Saturation3/1 -> [u_lqr]
  [switch] -> Enabled and Triggered Subsystem/Enable
  Constant6/1 -> Enabled and Triggered Subsystem/1(In1)
  Add4/1 -> MATLAB Function10/3(q2), MATLAB Function11/1(q2)
  [q2] -> Add4/1
  [q2_dot] -> MATLAB Function11/2(q2_dot)
  [k2] -> Add4/2
  Constant18/1 -> MATLAB Function10/7(kd)
  Constant19/1 -> MATLAB Function10/8(q1d)
  MATLAB Function11/1(u22) -> Saturation6/1
  Constant16/1 -> MATLAB Function11/3(k)
  MATLAB Function10/1(u) -> Saturation7/1
  [q1_dot] -> MATLAB Function10/2(q1_dot)
  Constant17/1 -> MATLAB Function10/6(kp)
  [q2_dot] -> MATLAB Function10/4(q2_dot)
  Saturation7/1 -> [u_swing]
  Saturation6/1 -> MATLAB Function10/5(u22)
  [q1] -> MATLAB Function10/1(q1)
  Saturation/1 -> [u_state], Abs/1, MATLAB Function/1(u)
  [k2] -> Add5/2
  [q2] -> Add5/1
  [q2] -> MATLAB Function3/1(q2)
  Mux1/1 -> Gain1/1
  Gain1/1 -> Saturation3/1
  [u_lqr] -> Switch/1
  Enabled and Triggered Subsystem/1(Out1) -> Switch/2
  Encoder PENDULUM/2 -> cobvert_encoder_2/1(In1)
  Encoder DC/2 -> convert_encoder/1(In1)
  convert_encoder/1(Out1) -> [q1]
  convert_encoder/2(Out2) -> [q1_dot]
  cobvert_encoder_2/1(Out1) -> [q2]
  cobvert_encoder_2/2(Out2) -> [q2_dot]
  Demux/1 -> Basic PWM/1
  Demux/2 -> Basic PWM/2
  Switch2/1 -> Demux/1
  Mux/1 -> Switch2/1
  Mux2/1 -> Switch2/3
  MATLAB Function/1(y) -> Switch2/2
  Constant4/1 -> Mux2/1
  Constant3/1 -> Mux/2
  Data Type Conversion/1 -> Mux2/2, Mux/1
  [u] -> Switch1/1
  Data Type Conversion2/1 -> UART Tx/6
  Constant5/1 -> Digital Output1/1
  [q1] -> Mux1/1
  [q1_dot] -> Mux1/2
  Add5/1 -> Mux1/3
  [q2_dot] -> Mux1/4
  [u_swing] -> Switch/3
  Digital Clock/1 -> Data Type Conversion2/1

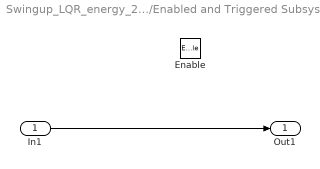
== system Swingup_LQR_energy_2021/Enabled and Triggered Subsystem ==
  In1 : Inport
  Enable : EnablePort
  Out1 : Outport  VectorParamsAs1DForOutWhenUnconnected=off
  wires:
  In1/1 -> Out1/1

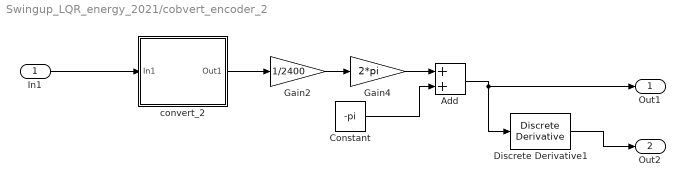
== system Swingup_LQR_energy_2021/cobvert_encoder_2 ==
  In1 : Inport
  Add : Sum
  Constant : Constant  Value=-pi  SampleTime=0.02
  Discrete Derivative1 : simulink/Discrete/Discrete Derivative  gainval=1.0  ICPrevScaledInput=0.0  OutMin=[]  OutMax=[]  OutDataType=fixdt(1, 16)  OutScaling=2^-10  DoSatur=off
  Gain2 : Gain  Gain=1/2400
  Gain4 : Gain  Gain=2*pi
  convert_2 : Subsystem
  Out1 : Outport  VectorParamsAs1DForOutWhenUnconnected=off
  Out2 : Outport  Port=2  VectorParamsAs1DForOutWhenUnconnected=off
  wires:
  Gain4/1 -> Add/1
  Constant/1 -> Add/2
  Add/1 -> Out1/1, Discrete Derivative1/1
  In1/1 -> convert_2/1(In1)
  convert_2/1(Out1) -> Gain2/1
  Discrete Derivative1/1 -> Out2/1
  Gain2/1 -> Gain4/1

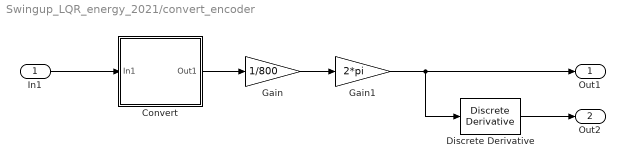
== system Swingup_LQR_energy_2021/convert_encoder ==
  In1 : Inport
  Convert : Subsystem
  Discrete Derivative : simulink/Discrete/Discrete Derivative  gainval=1.0  ICPrevScaledInput=0.0  OutMin=[]  OutMax=[]  OutDataType=fixdt(1, 16)  OutScaling=2^-10  DoSatur=off
  Gain : Gain  Gain=1/800
  Gain1 : Gain  Gain=2*pi
  Out1 : Outport  VectorParamsAs1DForOutWhenUnconnected=off
  Out2 : Outport  Port=2  VectorParamsAs1DForOutWhenUnconnected=off
  wires:
  In1/1 -> Convert/1(In1)
  Discrete Derivative/1 -> Out2/1
  Convert/1(Out1) -> Gain/1
  Gain1/1 -> Discrete Derivative/1, Out1/1
  Gain/1 -> Gain1/1

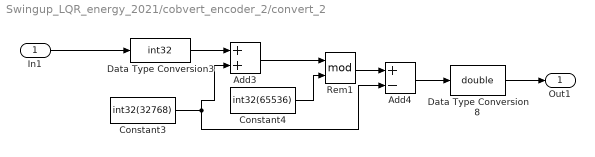
== system Swingup_LQR_energy_2021/cobvert_encoder_2/convert_2 ==
  In1 : Inport
  Add3 : Sum
  Add4 : Sum  Inputs=+-
  Constant3 : Constant  Value=int32(32768)  SampleTime=0.02
  Constant4 : Constant  Value=int32(65536)  SampleTime=0.02
  Data Type Conversion3 : DataTypeConversion  OutDataTypeStr=int32
  Data Type Conversion8 : DataTypeConversion  OutDataTypeStr=double
  Rem1 : Math  Operator=mod  SignedPower=on  SaturateOnIntegerOverflow=on
  Out1 : Outport  VectorParamsAs1DForOutWhenUnconnected=off
  wires:
  In1/1 -> Data Type Conversion3/1
  Data Type Conversion3/1 -> Add3/1
  Add4/1 -> Data Type Conversion8/1
  Rem1/1 -> Add4/1
  Add3/1 -> Rem1/1
  Data Type Conversion8/1 -> Out1/1
  Constant4/1 -> Rem1/2
  Constant3/1 -> Add3/2, Add4/2

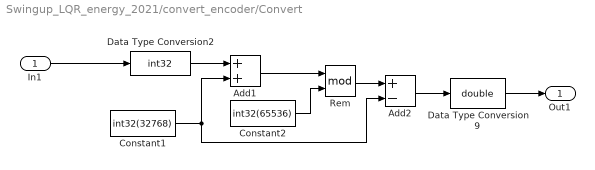
== system Swingup_LQR_energy_2021/convert_encoder/Convert ==
  In1 : Inport
  Add1 : Sum
  Add2 : Sum  Inputs=+-
  Constant1 : Constant  Value=int32(32768)  SampleTime=0.02
  Constant2 : Constant  Value=int32(65536)  SampleTime=0.02
  Data Type Conversion2 : DataTypeConversion  OutDataTypeStr=int32
  Data Type Conversion9 : DataTypeConversion  OutDataTypeStr=double
  Rem : Math  Operator=mod  SignedPower=on  SaturateOnIntegerOverflow=on
  Out1 : Outport  VectorParamsAs1DForOutWhenUnconnected=off
  wires:
  Add2/1 -> Data Type Conversion9/1
  Constant1/1 -> Add1/2, Add2/2
  Data Type Conversion9/1 -> Out1/1
  Add1/1 -> Rem/1
  Rem/1 -> Add2/1
  In1/1 -> Data Type Conversion2/1
  Constant2/1 -> Rem/2
  Data Type Conversion2/1 -> Add1/1

== matlab function Swingup_LQR_energy_2021/MATLAB Function ==
  data: u input; y output



function y= fcn(u)
if u>0
    y=0;
else
    y=1;
end

== matlab function Swingup_LQR_energy_2021/MATLAB Function3 ==
  data: q2 input; y output; q2_dot input; k2 output
function [y,k2]= fcn(q2,q2_dot)

k = round(q2/(2*pi));
k2 = k*2*pi;

if (abs(q2 - k*2*pi) < 0.3) && (abs(q2_dot) < 2)
    y = 1;
else
    y = 0;
end

== matlab function Swingup_LQR_energy_2021/MATLAB Function10 ==
  data: q1 input; u output; q1_dot input; q2 input; q2_dot input; u22 input; kp input; kd input; q1d input
function u = fcn(q1,q1_dot,q2,q2_dot,u22,kp,kd,q1d)

u = 0.9259*(0.09319*cos(q2)^2 - 0.4391)*(2.3*kd*q1_dot - 2.3*u22 + (2.3*(0.3143*q1_dot - 0.3928*sin(2.0*q2) - 1.0*q1_dot^2*(0.008641*sin(q2) - 0.008641*sin(q2)^3) + 0.01152*q2_dot^2*sin(q2) + 0.003142*q2_dot*cos(q2) - 0.003524*q1_dot*q2_dot*sin(2.0*q2)))/(0.02358*cos(q2)^2 - 0.1111) + 2.3*kp*(q1 - 1.0*q1d));

== matlab function Swingup_LQR_energy_2021/MATLAB Function11 ==
  data: q2 input; u22 output; q2_dot input; k input
function u22 = fcn(q2,q2_dot,k)


if q2_dot*cos(q2) == 0
    sig = 1;
else
    sig = sign(q2_dot*cos(q2));
end

u22 = -k*sig*((0.0036*q2_dot^2)/3 - 0.1650 + 0.1650*cos(q2));
